simulink model "Modelo_Grafico"  (R2015b)
settings: Solver=VariableStepAuto  StartTime=0  StopTime=15000  RelTol=1e-3
libraries: dspstat3 x2
settings Model: Creator=gmiglio  LastModifiedBy=gmiglio

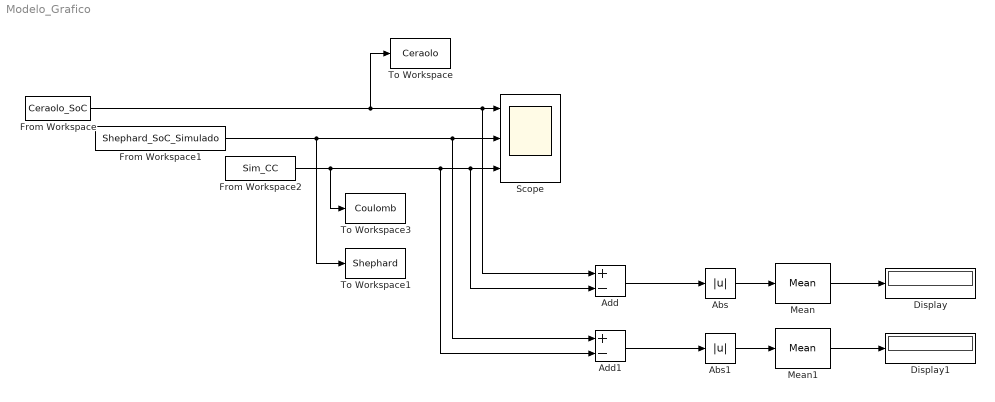
== system Modelo_Grafico ==
  Abs : Abs
  Abs1 : Abs
  Add : Sum  Inputs=+-
  Add1 : Sum  Inputs=+-
  Display : Display
      settings: Decimation=2
  Display1 : Display
      settings: Decimation=2
  From Workspace : FromWorkspace  VariableName=Ceraolo_SoC  SampleTime=0
  From Workspace1 : FromWorkspace  VariableName=Shephard_SoC_Simulado  SampleTime=0
  From Workspace2 : FromWorkspace  VariableName=Sim_CC  SampleTime=0
  Mean : dspstat3/Mean  run=off  reset_popup=None  InputProcessing=Columns as channels (frame based)  directionMode=Each column  dimension=1  roiEnable=off  roiType=Rectangles  roiPortion=Entire ROI  roiOutput=Individual statistics for each ROI  roiFlag=off  outputDataTypeStr=Inherit: Same as accumulator  outputLastDataTypeStr=Inherit: Same as accumulator  outputMin=[]  outputMax=[]  roundingMode=Floor  overflowMode=off
  Mean1 : dspstat3/Mean  run=off  reset_popup=None  InputProcessing=Columns as channels (frame based)  directionMode=Each column  dimension=1  roiEnable=off  roiType=Rectangles  roiPortion=Entire ROI  roiOutput=Individual statistics for each ROI  roiFlag=off  outputDataTypeStr=Inherit: Same as accumulator  outputLastDataTypeStr=Inherit: Same as accumulator  outputMin=[]  outputMax=[]  roundingMode=Floor  overflowMode=off
  Scope : Scope  NumInputPorts=3
  To Workspace : ToWorkspace  VariableName=Ceraolo  SaveFormat=Timeseries  SampleTime=-1
  To Workspace1 : ToWorkspace  VariableName=Shephard  SaveFormat=Timeseries  SampleTime=-1
  To Workspace3 : ToWorkspace  VariableName=Coulomb  SaveFormat=Timeseries  SampleTime=-1
  wires:
  From Workspace/1 -> To Workspace/1, Add/1, Scope/1
  From Workspace1/1 -> Add1/1, Scope/2, To Workspace1/1
  From Workspace2/1 -> Add1/2, Add/2, Scope/3, To Workspace3/1
  Add/1 -> Abs/1
  Add1/1 -> Abs1/1
  Abs/1 -> Mean/1
  Mean/1 -> Display/1
  Abs1/1 -> Mean1/1
  Mean1/1 -> Display1/1
